simulink model "verify_PumpAdditionalIntegrationSeries_mdl"  (R2018b)
settings: Solver=ode45  StartTime=0.0  StopTime=400  MaxStep=5  RelTol=1e-3  EnableMultiTasking=on
undefined symbols (not defined in the file or in its folder): path_carnot
libraries: carnot x5, simulink x4
settings Model: Creator=drhf  LastModifiedBy=drhf
settings DataIOCC: SaveFormat=Array  SignalLoggingSaveFormat=ModelDataLogs
settings OptimizationCC: ExpressionDepthLimit=2147483647  LifeSpan=inf
settings DebuggingCC: UnderspecifiedInitializationDetection=Classic  MergeDetectMultiDrivingBlocksExec=none  SolverPrmCheckMsg=warning  StateNameClashWarn=warning  SFUnexpectedBacktrackingDiag=warning  SFNoUnconditionalDefaultTransitionDiag=warning  SFExecutionAtInitializationDiag=none
settings HardwareCC: ProdBitPerPointer=32  ProdBitPerSizeT=32  ProdBitPerPtrDiffT=32  ProdLargestAtomicFloat=None  ProdIntDivRoundTo=Undefined  ProdEndianess=Unspecified  ProdWordSize=32  ProdHWDeviceType=32-bit Generic
settings ModelReferenceCC: PropagateSignalLabelsOutOfModel=off
settings SFSimCC: SimUseLocalCustomCode=off
settings RTWCC: RTWUseLocalCustomCode=off
settings CodeAppCC: StateflowObjectComments=on
settings GRTTargetCC: TargetLangStandard=C89/C90 (ANSI)  GeneratePreprocessorConditionals=Disable all  CombineOutputUpdateFcns=off  GRTInterface=on
settings ConfigComp: CovMetricSettings=dw  CovHtmlReporting=on  CovSaveCumulativeToWorkspaceVar=on  CovSaveSingleToWorkspaceVar=on  CovExternalEMLEnable=off

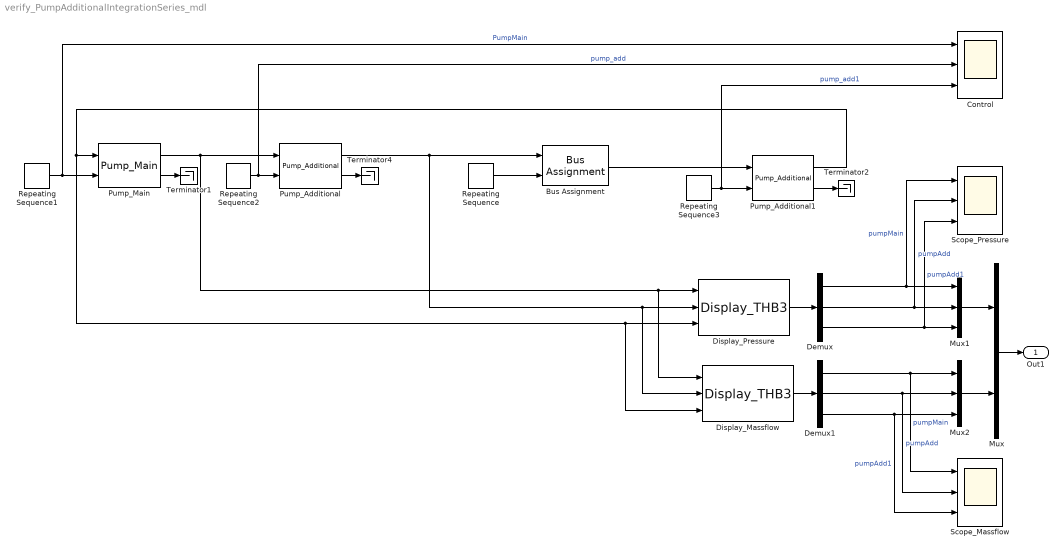
== system verify_PumpAdditionalIntegrationSeries_mdl ==
  Bus Assignment : BusAssignment  AssignedSignals=DPQuadratic
  Control : Scope  NumInputPorts=3
  Demux : Demux  Outputs=3
  Demux1 : Demux  Outputs=3
  Display_Massflow : carnot/Outputs/Display_THB3  t=off  m=on  p=off  id=off  mix=off  d=off
  Display_Pressure : carnot/Outputs/Display_THB3  t=off  m=off  p=on  id=off  mix=off  d=off
  Mux : Mux  Inputs=2
  Mux1 : Mux  Inputs=3
  Mux2 : Mux  Inputs=3
  Pump_Additional : carnot/Hydraulics/Pump_Additional  Tini=20  PathName=fullfile(path_carnot('libsl'), 'Hydraulics', 'Pump_Main', 'parameter_set')  FileName='Pump6m.mat'  userPath=off  userParam=off  a0=60000  a1=-43200  a2=0  dia=0.025  UA=1  mcp=4182  e0=50  e1=28.8  e2=-10.368
  Pump_Additional1 : carnot/Hydraulics/Pump_Additional  Tini=20  PathName=fullfile(path_carnot('libsl'), 'Hydraulics', 'Pump_Main', 'parameter_set')  FileName='Pump6m.mat'  userPath=off  userParam=off  a0=60000  a1=-43200  a2=0  dia=0.025  UA=1  mcp=4182  e0=50  e1=28.8  e2=-10.368
  Pump_Main : carnot/Hydraulics/Pump_Main  Tini=20  p0=3e5  IDpreset=pressure drop  fluid=Water  mix=0  mix2=0  mix3=0  t1=0.01  PathName=fullfile(path_carnot('libsl'), 'Hydraulics', 'Pump_Main', 'parameter_set')  FileName='Pump6m.mat'  userPath=off  userParam=off  a0=60000  a1=-43200  a2=0  dia=0.025  UA=1  mcp=4182  e0=50  e1=28.8  e2=-10.368
  Repeating Sequence : simulink/Sources/Repeating Sequence  rep_seq_t=[0 200 200.1 400]  rep_seq_y=[0 0 1 1]*(6e4/0.01)^2
  Repeating Sequence1 : simulink/Sources/Repeating Sequence  rep_seq_t=[0 150 180 200]  rep_seq_y=[1 1 0 0]
  Repeating Sequence2 : simulink/Sources/Repeating Sequence  rep_seq_t=[0 10 20 200]  rep_seq_y=[0 0 1 1]
  Repeating Sequence3 : simulink/Sources/Repeating Sequence  rep_seq_t=[0 40 40.1 50 60 200]  rep_seq_y=[1 1 0 0 1 1]
  Scope_Massflow : Scope  NumInputPorts=3
  Scope_Pressure : Scope  NumInputPorts=3
  Terminator1 : Terminator
  Terminator2 : Terminator
  Terminator4 : Terminator
  Out1 : Outport  SampleTime=5
  wires:
  Pump_Additional1/2 -> Terminator2/1
  Repeating Sequence1/1 -> Pump_Main/2, Control/1  "PumpMain"
  Bus Assignment/1 -> Pump_Additional1/1
  Display_Pressure/1 -> Demux/1
  Demux/1 -> Scope_Pressure/1, Mux1/1  "pumpMain"
  Demux/2 -> Mux1/2, Scope_Pressure/2  "pumpAdd"
  Demux/3 -> Scope_Pressure/3, Mux1/3  "pumpAdd1"
  Repeating Sequence3/1 -> Pump_Additional1/2, Control/3  "pump_add1"
  Pump_Main/2 -> Terminator1/1
  Repeating Sequence/1 -> Bus Assignment/2
  Pump_Main/1 -> Pump_Additional/1, Display_Massflow/1, Display_Pressure/1
  Pump_Additional/1 -> Bus Assignment/1, Display_Massflow/2, Display_Pressure/2
  Display_Massflow/1 -> Demux1/1
  Pump_Additional/2 -> Terminator4/1
  Repeating Sequence2/1 -> Control/2, Pump_Additional/2  "pump_add"
  Mux/1 -> Out1/1
  Demux1/1 -> Scope_Massflow/1, Mux2/1  "pumpMain"
  Demux1/2 -> Scope_Massflow/2, Mux2/2  "pumpAdd"
  Demux1/3 -> Mux2/3, Scope_Massflow/3  "pumpAdd1"
  Mux1/1 -> Mux/1
  Mux2/1 -> Mux/2
  Pump_Additional1/1 -> Display_Massflow/3, Display_Pressure/3, Pump_Main/1
